simulink model "Multicopter"  (R2018b)
settings: configuration reference "plant_config" (kept outside this file)
values from neighbouring files (symbols this model uses):
  PLANT_EXPORT = Simulink.Parameter(PLANT_EXPORT_VALUE)    [multicopter_model_init.m]    (also in plant_model_init.m)
undefined symbols (not defined in the file or in its folder): acc_x, acc_x_O, acc_y, acc_y_O, acc_z, acc_z_O, alt, alt_ref, day, DiscIntNeverNeededParam, fixType, flags, gSpeed, gyr_x, gyr_y, gyr_z, h_R, hAcc, headAcc, headMot, height, hMSL, hour, iTOW, lat, lat_ref, lon, lon_ref, M_BO, M_OB, mag_x, mag_y, mag_z, month, nano, Newton, numSV, pDOP, phi, PLANT_CONST, plant_model, pressure, prop_vel, psi, quat, Raphson, reserved1, reserved2, rot_x_B, rot_y_B, rot_z_B, sAcc, sec, Sensor_Model, tAcc, temperature, temprature, theta, timestamp, vAcc ... (+10)
libraries: simulink x6, dspsrcs4 x6, AP_Math x3, Rotation x2, Quaternion x2, aerolibatmos2 x1
(part 2 of 2)

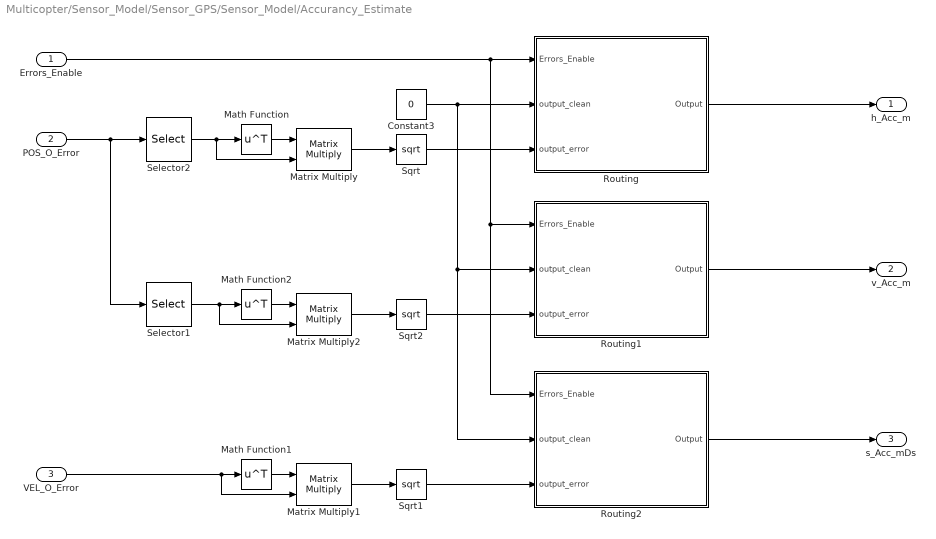
== system Multicopter/Sensor_Model/Sensor_GPS/Sensor_Model/Accurancy_Estimate ==
  Errors_Enable : Inport
  POS_O_Error : Inport  Port=2
  VEL_O_Error : Inport  Port=3
  Constant3 : Constant  Value=0
  Math Function : Math  Operator=transpose  SaturateOnIntegerOverflow=on
  Math Function1 : Math  Operator=transpose  SaturateOnIntegerOverflow=on
  Math Function2 : Math  Operator=transpose  SaturateOnIntegerOverflow=on
  Matrix Multiply : Product  Multiplication=Matrix(*)
  Matrix Multiply1 : Product  Multiplication=Matrix(*)
  Matrix Multiply2 : Product  Multiplication=Matrix(*)
  Routing : Subsystem
  Routing1 : Subsystem
  Routing2 : Subsystem
  Selector1 : Selector  InputPortWidth=3  IndexOptions=Index vector (dialog)  Indices=3  OutputSizes=1
  Selector2 : Selector  InputPortWidth=3  IndexOptions=Index vector (dialog)  Indices=[1 2]  OutputSizes=1
  Sqrt : Sqrt  OutputSignalType=real  SaturateOnIntegerOverflow=on
  Sqrt1 : Sqrt  OutputSignalType=real  SaturateOnIntegerOverflow=on
  Sqrt2 : Sqrt  OutputSignalType=real  SaturateOnIntegerOverflow=on
  h_Acc_m : Outport
  v_Acc_m : Outport  Port=2
  s_Acc_mDs : Outport  Port=3
  wires:
  Sqrt1/1 -> Routing2/3(output_error)
  Routing/1(Output) -> h_Acc_m/1
  Errors_Enable/1 -> Routing2/1(Errors_Enable), Routing1/1(Errors_Enable), Routing/1(Errors_Enable)
  POS_O_Error/1 -> Selector1/1, Selector2/1
  Sqrt/1 -> Routing/3(output_error)
  Constant3/1 -> Routing2/2(output_clean), Routing1/2(output_clean), Routing/2(output_clean)
  Routing1/1(Output) -> v_Acc_m/1
  Selector1/1 -> Math Function2/1, Matrix Multiply2/2
  Routing2/1(Output) -> s_Acc_mDs/1
  Math Function1/1 -> Matrix Multiply1/1
  Math Function2/1 -> Matrix Multiply2/1
  Math Function/1 -> Matrix Multiply/1
  Selector2/1 -> Matrix Multiply/2, Math Function/1
  Matrix Multiply1/1 -> Sqrt1/1
  Sqrt2/1 -> Routing1/3(output_error)
  Matrix Multiply/1 -> Sqrt/1
  Matrix Multiply2/1 -> Sqrt2/1
  VEL_O_Error/1 -> Matrix Multiply1/2, Math Function1/1

== system Multicopter/Sensor_Model/Sensor_GPS/Sensor_Model/GPS_Error ==
  Random Source : dspsrcs4/Random Source  SrcType=Gaussian  NormMethod=Ziggurat  CltLength=12  MinVal=0  MaxVal=1  MeanVal=0  VarVal=[0.02;0.02;0.04].^2  RepMode=Repeatable  rawSeed=1  IsInherit=off  SampMode=Discrete  SampTime=-1  SampFrame=1  DataType=Single  OutComplex=Real  OutputFrames=off
  Random Source1 : dspsrcs4/Random Source  SrcType=Gaussian  NormMethod=Ziggurat  CltLength=12  MinVal=0  MaxVal=1  MeanVal=0  VarVal=[0.01;0.01;0.01].^2  RepMode=Repeatable  rawSeed=1  IsInherit=off  SampMode=Discrete  SampTime=-1  SampFrame=1  DataType=Single  OutComplex=Real  OutputFrames=off
  POS_O_Error : Outport
  VEL_O_Error : Outport  Port=2
  wires:
  Random Source/1 -> POS_O_Error/1
  Random Source1/1 -> VEL_O_Error/1

== system Multicopter/Sensor_Model/Sensor_GPS/Sensor_Model/Routing ==
  Errors_Enable : Inport
  output_clean : Inport  Port=2
  output_error : Inport  Port=3
  Switch : Switch  Criteria=u2 > Threshold
  Output : Outport
  wires:
  output_clean/1 -> Switch/3
  output_error/1 -> Switch/1
  Errors_Enable/1 -> Switch/2
  Switch/1 -> Output/1

== system Multicopter/Sensor_Model/Sensor_GPS/Sensor_Model/Routing1 ==
  Errors_Enable : Inport
  output_clean : Inport  Port=2
  output_error : Inport  Port=3
  Switch : Switch  Criteria=u2 > Threshold
  Output : Outport
  wires:
  Switch/1 -> Output/1
  Errors_Enable/1 -> Switch/2
  output_error/1 -> Switch/1
  output_clean/1 -> Switch/3

== system Multicopter/Sensor_Model/Sensor_GPS/Sensor_Model/WGS84_Linearization ==
  POS_WGS84 : Inport
  POS_O_Error : Inport  Port=2
  Demux2 : Demux  Outputs=3
  Divide2 : Product  Inputs=/*
  Terminator2 : Terminator
  Vector Concatenate2 : Concatenate  NumInputs=3  Mode=Multidimensional array
  WGS84_Linearization : Subsystem  mask{a=6378137, f=1/298.257}
  POS_WGS84_Error : Outport
  wires:
  POS_WGS84/1 -> Demux2/1
  Demux2/1 -> WGS84_Linearization/1(mu_0)
  WGS84_Linearization/2(dy_dlambda) -> Vector Concatenate2/2
  POS_O_Error/1 -> Divide2/2
  Vector Concatenate2/1 -> Divide2/1
  WGS84_Linearization/1(dx_dmu) -> Vector Concatenate2/1
  Demux2/2 -> Terminator2/1
  Demux2/3 -> WGS84_Linearization/2(h_0)
  WGS84_Linearization/3(dz_dh) -> Vector Concatenate2/3
  Divide2/1 -> POS_WGS84_Error/1

== system Multicopter/Sensor_Model/Sensor_GPS/Sensor_Model/pos_filter ==
  POS_WGS84 : Inport
  Discrete FIR Filter : DiscreteFir
  POS_WGS84_meas : Outport
  wires:
  Discrete FIR Filter/1 -> POS_WGS84_meas/1
  POS_WGS84/1 -> Discrete FIR Filter/1

== system Multicopter/Sensor_Model/Sensor_GPS/Sensor_Model/vel_filter ==
  VEL_O : Inport
  Discrete FIR Filter : DiscreteFir
  VEL_O_meas : Outport
  wires:
  Discrete FIR Filter/1 -> VEL_O_meas/1
  VEL_O/1 -> Discrete FIR Filter/1

== system Multicopter/Sensor_Model/Sensor_IMU/Accelerometer/Bus Assignment ==
  Output : Inport
  Bus Creator : BusCreator  Inputs=3
  Demux : Demux  Outputs=3
  Acc_Raw : Outport
  wires:
  Demux/2 -> Bus Creator/2  "Acc_y_mDs2"
  Demux/3 -> Bus Creator/3  "Acc_z_mDs2"
  Demux/1 -> Bus Creator/1  "Acc_x_mDs2"
  Bus Creator/1 -> Acc_Raw/1
  Output/1 -> Demux/1

== system Multicopter/Sensor_Model/Sensor_IMU/Accelerometer/Physical_Model ==
  States : Inport
  Vibration_Enbale : Inport  Port=2
  Routing : Subsystem
  Specific_Force : Subsystem
  Sum1 : Sum  Inputs=|++
  Vibration_Model : Subsystem  TreatAsAtomicUnit=on  mask{Weight=Sensor_Model.Acc.Vibration.Weight, u_max=Sensor_Model.Acc.Vibration.RPM_Max, Gain=Sensor_Model.Acc.Vibration.Gain}
      mask prompts: Weight "input weight"; u_max "max RPM"; Gain "vibration gain"
      mask help: propeller vibration model
      settings: RTWSystemCode=Inline
  prop_vel : Subsystem
  sfor_B_mPs2 : Outport  Unit=m/s^2
  wires:
  States/1 -> prop_vel/1(States), Specific_Force/1(States)
  Routing/1(y) -> sfor_B_mPs2/1
  Sum1/1 -> Routing/3(output_error)
  Vibration_Model/1(vibration) -> Sum1/2
  Vibration_Enbale/1 -> Routing/1(Vibration_Enbale)
  prop_vel/1(omega_radDs) -> Vibration_Model/1(prop_rot_radPs)
  Specific_Force/1(sfor_B_mPs2) -> Routing/2(output_clean), Sum1/1

== system Multicopter/Sensor_Model/Sensor_IMU/Accelerometer/Sensor_Model ==
  Errors_Enables : Inport
  u : Inport  Port=2
  Lowpass_Filter : Subsystem
  Routing : Subsystem
  Saturation : Saturate  UpperLimit=Sensor_Model.Acc.Upper_limit  LowerLimit=Sensor_Model.Acc.Lower_limit
  Sensor_Error : Subsystem
  Sum : Sum  Inputs=|++
  White Noise : Subsystem
  y : Outport
  wires:
  Routing/1(y) -> y/1
  Errors_Enables/1 -> Routing/1(Errors_Enables)
  Sum/1 -> Routing/3(output_error)
  Saturation/1 -> Sum/1
  Lowpass_Filter/1(y) -> Saturation/1
  Sensor_Error/1(y) -> Lowpass_Filter/1(u)
  White Noise/1(noise) -> Sum/2
  u/1 -> Routing/2(output_clean), Sensor_Error/1(u)

== system Multicopter/Sensor_Model/Sensor_IMU/Gyroscope/Bus Assignment ==
  Output : Inport
  Bus Creator : BusCreator  Inputs=3
  Demux : Demux  Outputs=3
  Gyro_Raw : Outport
  wires:
  Demux/1 -> Bus Creator/1  "Gyro_x_radDs"
  Demux/2 -> Bus Creator/2  "Gyro_y_radDs"
  Demux/3 -> Bus Creator/3  "Gyro_z_radDs"
  Bus Creator/1 -> Gyro_Raw/1
  Output/1 -> Demux/1

== system Multicopter/Sensor_Model/Sensor_IMU/Gyroscope/Physical_Model ==
  States : Inport
  Vibration_Enable : Inport  Port=2
  Routing : Subsystem
  Sum : Sum  Inputs=|++
  Vibration_Model : Subsystem  TreatAsAtomicUnit=on  mask{Weight=Sensor_Model.Gyro.Vibration.Weight, u_max=Sensor_Model.Gyro.Vibration.RPM_Max, Gain=Sensor_Model.Gyro.Vibration.Gain}
      mask prompts: Weight "input weight"; u_max "max RPM"; Gain "vibration gain"
      mask help: propeller vibration model
      settings: RTWSystemCode=Inline
  prop_vel : Subsystem
  selection : Subsystem
  gyr_B_radDs : Outport  Unit=rad/s
  wires:
  States/1 -> selection/1(States), prop_vel/1(States)
  selection/1(rot_radPs) -> Sum/1, Routing/2(output_clean)
  Sum/1 -> Routing/3(output_error)
  Vibration_Model/1(vibration) -> Sum/2
  Routing/1(y) -> gyr_B_radDs/1
  Vibration_Enable/1 -> Routing/1(Vibration_Enable)
  prop_vel/1(omega_radPs) -> Vibration_Model/1(prop_rot_radPs)

== system Multicopter/Sensor_Model/Sensor_IMU/Gyroscope/Sensor_Model ==
  Errors_Enable : Inport
  u : Inport  Port=2
  LPF : Subsystem
  Routing : Subsystem
  Saturation : Saturate  UpperLimit=Sensor_Model.Gyro.Range  LowerLimit=-Sensor_Model.Gyro.Range
  Sensor_Error : Subsystem
  Sum : Sum  Inputs=|++
  White Noise : Subsystem
  y : Outport
  wires:
  u/1 -> Routing/2(output_clean), Sensor_Error/1(u)
  Routing/1(y) -> y/1
  Errors_Enable/1 -> Routing/1(Errors_Enable)
  Sum/1 -> Routing/3(output_error)
  Saturation/1 -> Sum/1
  LPF/1(y) -> Saturation/1
  Sensor_Error/1(y) -> LPF/1(u)
  White Noise/1(noise) -> Sum/2

== system Multicopter/Sensor_Model/Sensor_MAG/Sensor_Magnetometer/Bus Assignment ==
  Output : Inport
  Bus Creator : BusCreator  Inputs=3
  Demux : Demux  Outputs=3
  Mag_Raw : Outport
  wires:
  Demux/2 -> Bus Creator/2  "Mag_y_gauss"
  Demux/1 -> Bus Creator/1  "Mag_x_gauss"
  Bus Creator/1 -> Mag_Raw/1
  Demux/3 -> Bus Creator/3  "Mag_z_gauss"
  Output/1 -> Demux/1

== system Multicopter/Sensor_Model/Sensor_MAG/Sensor_Magnetometer/Physical_Model ==
  States : Inport
  Bus Selector : BusSelector  OutputSignals=Plant_States.lat,Plant_States.lon
  Bus Selector1 : BusSelector  OutputSignals=Extended_States.M_BO
  Magnetic_Field : Subsystem
  Product : Product  Multiplication=Matrix(*)  RndMeth=Zero  InputSameDT=on  OutDataTypeStr=Inherit: Same as first input
  wmm_lookup : Subsystem  mask{wmm_magnitude=Sensor_Model.Mag.WMM_Mag, wmm_declination=Sensor_Model.Mag.WMM_Dec, wmm_inclination=Sensor_Model.Mag.WMM_Inc, res=10}
      mask prompts: wmm_magnitude "WMM Magnitude Lookup Table"; wmm_declination "WMM Declination Lookup Table"; wmm_inclination "WMM Inclination Lookup Table"; res "Resolution"
  mag_B_Gauss : Outport  Unit=T  PortDimensions=[3 1]
  wires:
  States/1 -> Bus Selector1/1, Bus Selector/1
  Bus Selector/2 -> wmm_lookup/2(lon_rad)  "<lon>"
  Bus Selector/1 -> wmm_lookup/1(lat_rad)  "<lat>"
  wmm_lookup/1(magnitude_uT) -> Magnetic_Field/1(magnitude_uT)
  wmm_lookup/2(declination_deg) -> Magnetic_Field/2(declination_deg)
  wmm_lookup/3(inclination_deg) -> Magnetic_Field/3(inclination_deg)
  Bus Selector1/1 -> Product/1  "<M_BO>"
  Product/1 -> mag_B_Gauss/1
  Magnetic_Field/1(mag_O_gauss) -> Product/2

== system Multicopter/Sensor_Model/Sensor_MAG/Sensor_Magnetometer/Sensor_Model ==
  Errors_Enable : Inport
  u : Inport  Port=2
  Add : Sum  InputSameDT=on  OutDataTypeStr=Inherit: Same as first input
  Routing : Subsystem
  Saturation : Saturate  UpperLimit=Sensor_Model.Mag.Upper_limit  LowerLimit=Sensor_Model.Mag.Lower_limit
  Sensor_Error : Subsystem
  Signal Conversion1 : SignalConversion  OverrideOpt=on
  White_Noise : Subsystem
  y : Outport
  wires:
  Signal Conversion1/1 -> Routing/2(output_clean)
  Routing/1(y) -> y/1
  Errors_Enable/1 -> Routing/1(Errors_Enable)
  Add/1 -> Routing/3(output_error)
  Saturation/1 -> Add/1
  Sensor_Error/1(y) -> Saturation/1
  u/1 -> Signal Conversion1/1, Sensor_Error/1(u)
  White_Noise/1(noise) -> Add/2

== system Multicopter/Sensor_Model/Sensor_GPS/Sensor_Model/Accurancy_Estimate/Routing ==
  Errors_Enable : Inport
  output_clean : Inport  Port=2
  output_error : Inport  Port=3
  Switch : Switch  Criteria=u2 > Threshold
  Output : Outport
  wires:
  output_clean/1 -> Switch/3
  output_error/1 -> Switch/1
  Errors_Enable/1 -> Switch/2
  Switch/1 -> Output/1

== system Multicopter/Sensor_Model/Sensor_GPS/Sensor_Model/Accurancy_Estimate/Routing1 ==
  Errors_Enable : Inport
  output_clean : Inport  Port=2
  output_error : Inport  Port=3
  Switch : Switch  Criteria=u2 > Threshold
  Output : Outport
  wires:
  Switch/1 -> Output/1
  Errors_Enable/1 -> Switch/2
  output_error/1 -> Switch/1
  output_clean/1 -> Switch/3

== system Multicopter/Sensor_Model/Sensor_GPS/Sensor_Model/Accurancy_Estimate/Routing2 ==
  Errors_Enable : Inport
  output_clean : Inport  Port=2
  output_error : Inport  Port=3
  Switch : Switch  Criteria=u2 > Threshold
  Output : Outport
  wires:
  output_clean/1 -> Switch/3
  output_error/1 -> Switch/1
  Errors_Enable/1 -> Switch/2
  Switch/1 -> Output/1

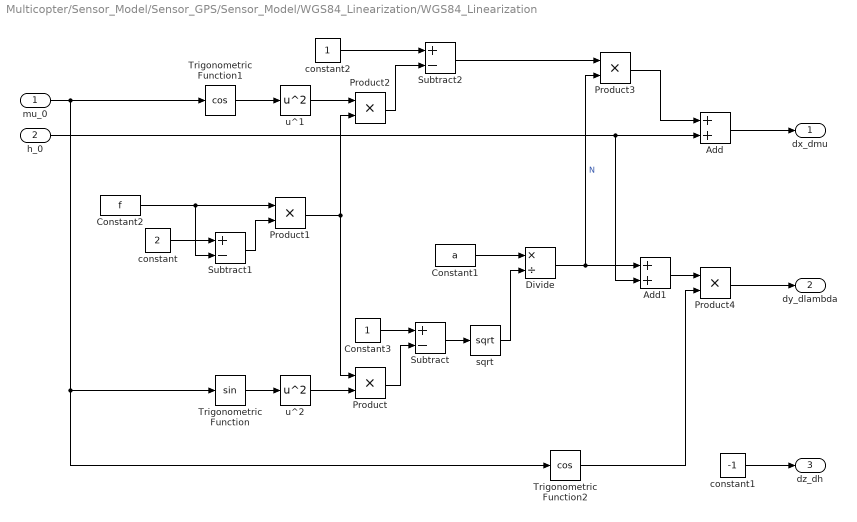
== system Multicopter/Sensor_Model/Sensor_GPS/Sensor_Model/WGS84_Linearization/WGS84_Linearization ==
  mu_0 : Inport
  h_0 : Inport  Port=2
  Add : Sum
  Add1 : Sum
  Constant1 : Constant  Value=a
  Constant2 : Constant  Value=f
  Constant3 : Constant
  Divide : Product  Inputs=*/
  Product{,1..4} (5 alike) : Product  RndMeth=Zero
  Subtract : Sum  Inputs=+-
  Subtract1 : Sum  Inputs=+-
  Subtract2 : Sum  Inputs=+-
  Trigonometric Function : Trigonometry
  Trigonometric Function1 : Trigonometry  Operator=cos
  Trigonometric Function2 : Trigonometry  Operator=cos
  constant : Constant  Value=2
  constant1 : Constant  Value=-1
  constant2 : Constant
  sqrt : Sqrt  AlgorithmType=Newton-Raphson  SaturateOnIntegerOverflow=on
  u^1 : Math  Operator=square  SaturateOnIntegerOverflow=on
  u^2 : Math  Operator=square  SaturateOnIntegerOverflow=on
  dx_dmu : Outport
  dy_dlambda : Outport  Port=2
  dz_dh : Outport  Port=3
  wires:
  Product4/1 -> dy_dlambda/1
  Add1/1 -> Product4/1
  Trigonometric Function2/1 -> Product4/2
  Product3/1 -> Add/1
  Subtract2/1 -> Product3/1
  Product2/1 -> Subtract2/2
  u^1/1 -> Product2/1
  Trigonometric Function1/1 -> u^1/1
  constant2/1 -> Subtract2/1
  h_0/1 -> Add1/2, Add/2
  Add/1 -> dx_dmu/1
  constant1/1 -> dz_dh/1
  Divide/1 -> Add1/1, Product3/2  "N"
  sqrt/1 -> Divide/2
  Product1/1 -> Product2/2, Product/1
  Subtract1/1 -> Product1/2
  constant/1 -> Subtract1/1
  Constant2/1 -> Subtract1/2, Product1/1
  Product/1 -> Subtract/2
  Subtract/1 -> sqrt/1
  Constant3/1 -> Subtract/1
  u^2/1 -> Product/2
  Trigonometric Function/1 -> u^2/1
  mu_0/1 -> Trigonometric Function2/1, Trigonometric Function/1, Trigonometric Function1/1
  Constant1/1 -> Divide/1

== system Multicopter/Sensor_Model/Sensor_IMU/Accelerometer/Physical_Model/Routing ==
  Vibration_Enbale : Inport
  output_clean : Inport  Port=2
  output_error : Inport  Port=3
  Switch : Switch  Criteria=u2 > Threshold  OutDataTypeStr=single
  y : Outport
  wires:
  Vibration_Enbale/1 -> Switch/2
  output_clean/1 -> Switch/3
  output_error/1 -> Switch/1
  Switch/1 -> y/1

== system Multicopter/Sensor_Model/Sensor_IMU/Accelerometer/Physical_Model/Specific_Force ==
  States : Inport
  Bus Selector : BusSelector  OutputSignals=Plant_States.acc_x_O,Plant_States.acc_y_O,Plant_States.acc_z_O
  Bus Selector1 : BusSelector  OutputSignals=Extended_States.M_BO
  Gravity : Constant  Value=[0;0;Sensor_Model.g]  OutDataTypeStr=single
  Product1 : Product  Multiplication=Matrix(*)  RndMeth=Zero  InputSameDT=on  OutDataTypeStr=Inherit: Same as first input
  Sum : Sum  Inputs=|+-  InputSameDT=on  OutDataTypeStr=Inherit: Same as first input
  Vector Concatenate1 : Concatenate  NumInputs=3  Mode=Multidimensional array
  sfor_B_mPs2 : Outport  Unit=m/s^2
  wires:
  States/1 -> Bus Selector1/1, Bus Selector/1
  Bus Selector/1 -> Vector Concatenate1/1  "<acc_x_O>"
  Bus Selector/2 -> Vector Concatenate1/2  "<acc_y_O>"
  Bus Selector/3 -> Vector Concatenate1/3  "<acc_z_O>"
  Product1/1 -> sfor_B_mPs2/1
  Bus Selector1/1 -> Product1/1  "<M_BO>"
  Vector Concatenate1/1 -> Sum/1
  Sum/1 -> Product1/2
  Gravity/1 -> Sum/2

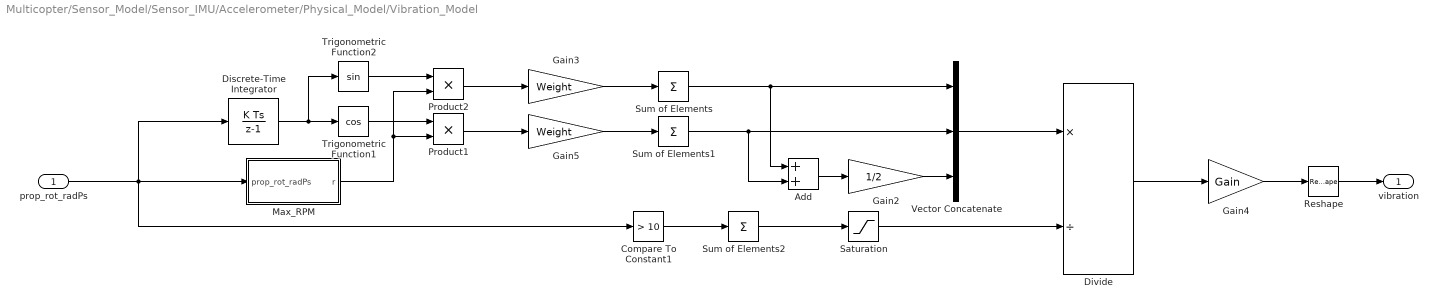
== system Multicopter/Sensor_Model/Sensor_IMU/Accelerometer/Physical_Model/Vibration_Model ==
  prop_rot_radPs : Inport  PortDimensions=[4,1]
  Add : Sum
  Compare To Constant1 : simulink/Logic and Bit Operations/Compare To Constant  relop=>  const=10  OutDataTypeStr=boolean
  Discrete-Time Integrator : DiscreteIntegrator  InitialCondition=zeros(4,1)  SampleTime=-1  ICPrevOutput=DiscIntNeverNeededParam  ICPrevScaledInput=DiscIntNeverNeededParam
  Divide : Product  Inputs=*/
  Gain2 : Gain  Gain=1/2
  Gain3 : Gain  Gain=Weight
  Gain4 : Gain  Gain=Gain
  Gain5 : Gain  Gain=Weight
  Max_RPM : Subsystem
  Product1 : Product  RndMeth=Zero
  Product2 : Product  RndMeth=Zero
  Reshape : Reshape  OutputDimensionality=Column vector (2-D)
  Saturation : Saturate  UpperLimit=8  LowerLimit=4
  Sum of Elements : Sum  Inputs=+
  Sum of Elements1 : Sum  Inputs=+
  Sum of Elements2 : Sum  Inputs=+  CollapseMode=Specified dimension
  Trigonometric Function1 : Trigonometry  Operator=cos
  Trigonometric Function2 : Trigonometry
  Vector Concatenate : Concatenate  NumInputs=3  Mode=Multidimensional array
  vibration : Outport
  wires:
  prop_rot_radPs/1 -> Discrete-Time Integrator/1, Compare To Constant1/1, Max_RPM/1(prop_rot_radPs)
  Sum of Elements2/1 -> Saturation/1
  Saturation/1 -> Divide/2
  Divide/1 -> Gain4/1
  Compare To Constant1/1 -> Sum of Elements2/1
  Vector Concatenate/1 -> Divide/1
  Product1/1 -> Gain5/1
  Trigonometric Function1/1 -> Product1/1
  Product2/1 -> Gain3/1
  Trigonometric Function2/1 -> Product2/1
  Gain2/1 -> Vector Concatenate/3
  Add/1 -> Gain2/1
  Sum of Elements1/1 -> Add/2, Vector Concatenate/2
  Discrete-Time Integrator/1 -> Trigonometric Function2/1, Trigonometric Function1/1
  Sum of Elements/1 -> Add/1, Vector Concatenate/1
  Reshape/1 -> vibration/1
  Gain3/1 -> Sum of Elements/1
  Gain5/1 -> Sum of Elements1/1
  Gain4/1 -> Reshape/1
  Max_RPM/1(r) -> Product1/2, Product2/2

== system Multicopter/Sensor_Model/Sensor_IMU/Accelerometer/Physical_Model/prop_vel ==
  States : Inport
  Bus Selector2 : BusSelector  OutputSignals=Extended_States.prop_vel
  Selector : Selector  InputPortWidth=8  IndexOptions=Index vector (dialog)  Indices=[1:4]  OutputSizes=1
  omega_radDs : Outport
  wires:
  States/1 -> Bus Selector2/1
  Bus Selector2/1 -> Selector/1  "<prop_vel>"
  Selector/1 -> omega_radDs/1

== system Multicopter/Sensor_Model/Sensor_IMU/Accelerometer/Sensor_Model/Lowpass_Filter ==
  u : Inport
  Constant : Constant  Value=2*pi*Sensor_Model.Acc.Cutoff_frequency_Hz  VectorParams1D=off  OutDataTypeStr=single
  Product : Product  RndMeth=Zero  InputSameDT=on  OutDataTypeStr=Inherit: Same as first input
  Product1 : Product  RndMeth=Zero  InputSameDT=on  OutDataTypeStr=Inherit: Same as first input
  Sum : Sum  Inputs=|+-  InputSameDT=on  OutDataTypeStr=Inherit: Same as first input
  Sum1 : Sum  Inputs=|+-  InputSameDT=on  OutDataTypeStr=Inherit: Same as first input
  integrate : DiscreteIntegrator  SampleTime=-1  ICPrevOutput=DiscIntNeverNeededParam  ICPrevScaledInput=DiscIntNeverNeededParam
  integrate1 : DiscreteIntegrator  SampleTime=-1  ICPrevOutput=DiscIntNeverNeededParam  ICPrevScaledInput=DiscIntNeverNeededParam
  y : Outport
  wires:
  integrate1/1 -> Sum1/2, y/1
  Product1/1 -> integrate1/1
  Sum1/1 -> Product1/2
  integrate/1 -> Sum/2, Sum1/1
  Product/1 -> integrate/1
  Constant/1 -> Product1/1, Product/1
  Sum/1 -> Product/2
  u/1 -> Sum/1

== system Multicopter/Sensor_Model/Sensor_IMU/Accelerometer/Sensor_Model/Routing ==
  Errors_Enables : Inport
  output_clean : Inport  Port=2
  output_error : Inport  Port=3
  Switch : Switch  Criteria=u2 > Threshold
  y : Outport
  wires:
  Switch/1 -> y/1
  output_error/1 -> Switch/1
  output_clean/1 -> Switch/3
  Errors_Enables/1 -> Switch/2

== system Multicopter/Sensor_Model/Sensor_IMU/Accelerometer/Sensor_Model/Sensor_Error ==
  u : Inport
  Add : Sum  InputSameDT=on  OutDataTypeStr=Inherit: Same as first input
  Constant : Constant  Value=eye(3)  OutDataTypeStr=single
  Constant1 : Constant  Value=Sensor_Model.Acc.Scalefactor_Error  VectorParams1D=off  OutDataTypeStr=single
  Constant3 : Constant  Value=Sensor_Model.Acc.Bias  VectorParams1D=off  OutDataTypeStr=single
  Product : Product  Multiplication=Matrix(*)  RndMeth=Zero  InputSameDT=on  OutDataTypeStr=Inherit: Same as first input
  Sum : Sum  Inputs=|++  InputSameDT=on  OutDataTypeStr=Inherit: Same as first input
  y : Outport
  wires:
  Sum/1 -> y/1
  Add/1 -> Product/1
  u/1 -> Product/2
  Constant1/1 -> Add/2
  Constant/1 -> Add/1
  Product/1 -> Sum/1
  Constant3/1 -> Sum/2

== system Multicopter/Sensor_Model/Sensor_IMU/Accelerometer/Sensor_Model/White Noise ==
  Random Source : dspsrcs4/Random Source  SrcType=Gaussian  NormMethod=Ziggurat  CltLength=12  MinVal=0  MaxVal=1  MeanVal=0  VarVal=Sensor_Model.Acc.Variance  RepMode=Repeatable  rawSeed=1  IsInherit=off  SampMode=Discrete  SampTime=-1  SampFrame=1  DataType=Single  OutComplex=Real  OutputFrames=off
  noise : Outport
  wires:
  Random Source/1 -> noise/1

== system Multicopter/Sensor_Model/Sensor_IMU/Gyroscope/Physical_Model/Routing ==
  Vibration_Enable : Inport
  output_clean : Inport  Port=2
  output_error : Inport  Port=3
  Switch : Switch  Criteria=u2 > Threshold
  y : Outport
  wires:
  Vibration_Enable/1 -> Switch/2
  output_clean/1 -> Switch/3
  output_error/1 -> Switch/1
  Switch/1 -> y/1

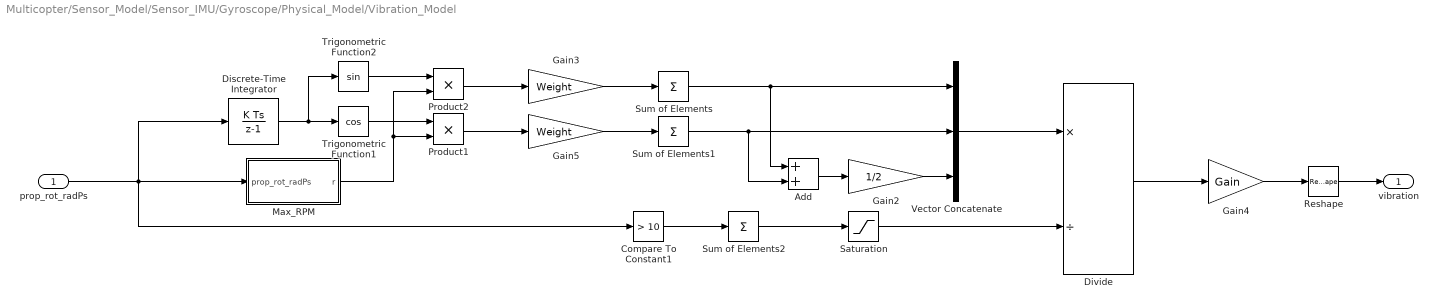
== system Multicopter/Sensor_Model/Sensor_IMU/Gyroscope/Physical_Model/Vibration_Model ==
  prop_rot_radPs : Inport  PortDimensions=[4,1]
  Add : Sum
  Compare To Constant1 : simulink/Logic and Bit Operations/Compare To Constant  relop=>  const=10  OutDataTypeStr=boolean
  Discrete-Time Integrator : DiscreteIntegrator  InitialCondition=zeros(4,1)  SampleTime=-1  ICPrevOutput=DiscIntNeverNeededParam  ICPrevScaledInput=DiscIntNeverNeededParam
  Divide : Product  Inputs=*/
  Gain2 : Gain  Gain=1/2
  Gain3 : Gain  Gain=Weight
  Gain4 : Gain  Gain=Gain
  Gain5 : Gain  Gain=Weight
  Max_RPM : Subsystem
  Product1 : Product  RndMeth=Zero
  Product2 : Product  RndMeth=Zero
  Reshape : Reshape  OutputDimensionality=Column vector (2-D)
  Saturation : Saturate  UpperLimit=8  LowerLimit=4
  Sum of Elements : Sum  Inputs=+
  Sum of Elements1 : Sum  Inputs=+
  Sum of Elements2 : Sum  Inputs=+  CollapseMode=Specified dimension
  Trigonometric Function1 : Trigonometry  Operator=cos
  Trigonometric Function2 : Trigonometry
  Vector Concatenate : Concatenate  NumInputs=3  Mode=Multidimensional array
  vibration : Outport
  wires:
  prop_rot_radPs/1 -> Discrete-Time Integrator/1, Compare To Constant1/1, Max_RPM/1(prop_rot_radPs)
  Sum of Elements2/1 -> Saturation/1
  Saturation/1 -> Divide/2
  Divide/1 -> Gain4/1
  Compare To Constant1/1 -> Sum of Elements2/1
  Vector Concatenate/1 -> Divide/1
  Product1/1 -> Gain5/1
  Trigonometric Function1/1 -> Product1/1
  Product2/1 -> Gain3/1
  Trigonometric Function2/1 -> Product2/1
  Gain2/1 -> Vector Concatenate/3
  Add/1 -> Gain2/1
  Sum of Elements1/1 -> Add/2, Vector Concatenate/2
  Discrete-Time Integrator/1 -> Trigonometric Function2/1, Trigonometric Function1/1
  Sum of Elements/1 -> Add/1, Vector Concatenate/1
  Reshape/1 -> vibration/1
  Gain3/1 -> Sum of Elements/1
  Gain5/1 -> Sum of Elements1/1
  Gain4/1 -> Reshape/1
  Max_RPM/1(r) -> Product1/2, Product2/2

== system Multicopter/Sensor_Model/Sensor_IMU/Gyroscope/Physical_Model/prop_vel ==
  States : Inport
  Bus Selector2 : BusSelector  OutputSignals=Extended_States.prop_vel
  Selector : Selector  InputPortWidth=8  IndexOptions=Index vector (dialog)  Indices=[1:4]  OutputSizes=1
  omega_radPs : Outport
  wires:
  Selector/1 -> omega_radPs/1
  States/1 -> Bus Selector2/1
  Bus Selector2/1 -> Selector/1  "<prop_vel>"

== system Multicopter/Sensor_Model/Sensor_IMU/Gyroscope/Physical_Model/selection ==
  States : Inport
  Bus Selector2 : BusSelector  OutputSignals=Plant_States.rot_x_B,Plant_States.rot_y_B,Plant_States.rot_z_B
  Vector Concatenate : Concatenate  NumInputs=3  Mode=Multidimensional array
  rot_radPs : Outport
  wires:
  Vector Concatenate/1 -> rot_radPs/1
  Bus Selector2/3 -> Vector Concatenate/3  "<rot_z_B>"
  Bus Selector2/1 -> Vector Concatenate/1  "<rot_x_B>"
  Bus Selector2/2 -> Vector Concatenate/2  "<rot_y_B>"
  States/1 -> Bus Selector2/1

== system Multicopter/Sensor_Model/Sensor_IMU/Gyroscope/Sensor_Model/LPF ==
  u : Inport
  Constant : Constant  Value=2*pi*Sensor_Model.Gyro.Cutoff_frequency_Hz  VectorParams1D=off  OutDataTypeStr=single
  Product : Product  RndMeth=Zero  InputSameDT=on  OutDataTypeStr=Inherit: Same as first input
  Product1 : Product  RndMeth=Zero  InputSameDT=on  OutDataTypeStr=Inherit: Same as first input
  Sum : Sum  Inputs=|+-  InputSameDT=on  OutDataTypeStr=Inherit: Same as first input
  Sum1 : Sum  Inputs=|+-  InputSameDT=on  OutDataTypeStr=Inherit: Same as first input
  integrate : DiscreteIntegrator  SampleTime=-1  ICPrevOutput=DiscIntNeverNeededParam  ICPrevScaledInput=DiscIntNeverNeededParam
  integrate1 : DiscreteIntegrator  SampleTime=-1  ICPrevOutput=DiscIntNeverNeededParam  ICPrevScaledInput=DiscIntNeverNeededParam
  y : Outport
  wires:
  integrate1/1 -> Sum1/2, y/1
  Product1/1 -> integrate1/1
  Sum1/1 -> Product1/2
  integrate/1 -> Sum/2, Sum1/1
  Product/1 -> integrate/1
  Constant/1 -> Product1/1, Product/1
  Sum/1 -> Product/2
  u/1 -> Sum/1

== system Multicopter/Sensor_Model/Sensor_IMU/Gyroscope/Sensor_Model/Routing ==
  Errors_Enable : Inport
  output_clean : Inport  Port=2
  output_error : Inport  Port=3
  Switch : Switch  Criteria=u2 > Threshold
  y : Outport
  wires:
  Switch/1 -> y/1
  output_error/1 -> Switch/1
  output_clean/1 -> Switch/3
  Errors_Enable/1 -> Switch/2

== system Multicopter/Sensor_Model/Sensor_IMU/Gyroscope/Sensor_Model/Sensor_Error ==
  u : Inport
  Add : Sum  InputSameDT=on  OutDataTypeStr=Inherit: Same as first input
  Constant1 : Constant  Value=Sensor_Model.Gyro.Scalefactor_Error  VectorParams1D=off  OutDataTypeStr=single
  Constant2 : Constant  Value=eye(3)  OutDataTypeStr=single
  Constant3 : Constant  Value=Sensor_Model.Gyro.Bias  VectorParams1D=off  OutDataTypeStr=single
  Product : Product  Multiplication=Matrix(*)  RndMeth=Zero  InputSameDT=on  OutDataTypeStr=Inherit: Same as first input
  Sum : Sum  Inputs=|++  InputSameDT=on  OutDataTypeStr=Inherit: Same as first input
  y : Outport
  wires:
  Sum/1 -> y/1
  Product/1 -> Sum/1
  u/1 -> Product/2
  Add/1 -> Product/1
  Constant1/1 -> Add/2
  Constant2/1 -> Add/1
  Constant3/1 -> Sum/2

== system Multicopter/Sensor_Model/Sensor_IMU/Gyroscope/Sensor_Model/White Noise ==
  Random Source : dspsrcs4/Random Source  SrcType=Gaussian  NormMethod=Ziggurat  CltLength=12  MinVal=0  MaxVal=1  MeanVal=0  VarVal=Sensor_Model.Gyro.Variance  RepMode=Repeatable  rawSeed=1  IsInherit=off  SampMode=Discrete  SampTime=-1  SampFrame=1  DataType=Single  OutComplex=Real  OutputFrames=off
  noise : Outport
  wires:
  Random Source/1 -> noise/1

== system Multicopter/Sensor_Model/Sensor_MAG/Sensor_Magnetometer/Physical_Model/Magnetic_Field ==
  magnitude_uT : Inport
  declination_deg : Inport  Port=2
  inclination_deg : Inport  Port=3
  Constant : Constant  Value=[1;0;0]  OutDataTypeStr=single
  Gain : Gain  Gain=-pi/180
  Gain1 : Gain  Gain=pi/180
  Gain2 : Gain  Gain=0.01
  Multiply : Product
  Multiply1 : Product  Multiplication=Matrix(*)
  Multiply2 : Product  Multiplication=Matrix(*)
  Rot_y to M : Subsystem
  Rot_z to M : Subsystem
  mag_O_gauss : Outport
  wires:
  Constant/1 -> Multiply/2
  Multiply/1 -> Multiply1/2  "mag_field"
  Rot_y to M/1(My) -> Multiply1/1
  inclination_deg/1 -> Gain/1
  Gain/1 -> Rot_y to M/1(alpha)
  declination_deg/1 -> Gain1/1
  Gain1/1 -> Rot_z to M/1(alpha)
  Rot_z to M/1(Mz) -> Multiply2/1
  magnitude_uT/1 -> Gain2/1
  Gain2/1 -> Multiply/1  "magnitude_gauss"
  Multiply1/1 -> Multiply2/2
  Multiply2/1 -> mag_O_gauss/1

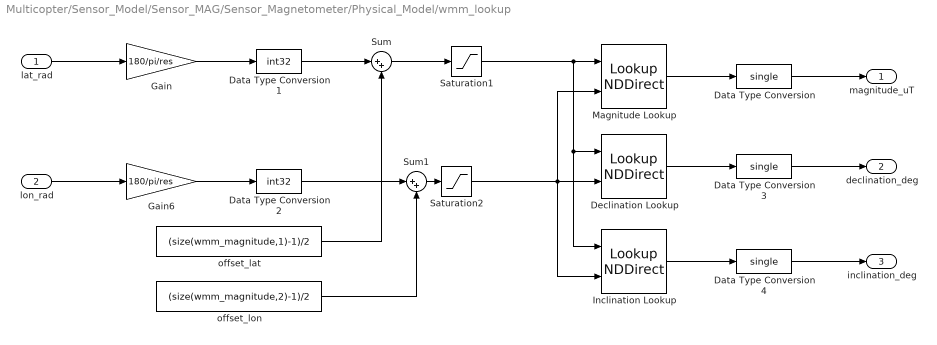
== system Multicopter/Sensor_Model/Sensor_MAG/Sensor_Magnetometer/Physical_Model/wmm_lookup ==
  lat_rad : Inport
  lon_rad : Inport  Port=2
  Data Type Conversion : DataTypeConversion  OutDataTypeStr=single
  Data Type Conversion1 : DataTypeConversion  OutDataTypeStr=int32  RndMeth=Simplest
  Data Type Conversion2 : DataTypeConversion  OutDataTypeStr=int32  RndMeth=Simplest
  Data Type Conversion3 : DataTypeConversion  OutDataTypeStr=single
  Data Type Conversion4 : DataTypeConversion  OutDataTypeStr=single
  Declination Lookup : LookupNDDirect  Table=wmm_declination  TableDataTypeStr=int16
  Gain : Gain  Gain=180/pi/res
  Gain6 : Gain  Gain=180/pi/res
  Inclination Lookup : LookupNDDirect  Table=wmm_inclination  TableDataTypeStr=int8
  Magnitude Lookup : LookupNDDirect  Table=wmm_magnitude  TableDataTypeStr=uint8
  Saturation1 : Saturate  UpperLimit=size(wmm_magnitude,1)-1  LowerLimit=0
  Saturation2 : Saturate  UpperLimit=size(wmm_magnitude,2)-1  LowerLimit=0
  Sum : Sum  Inputs=|++
  Sum1 : Sum  Inputs=|++
  offset_lat : Constant  Value=(size(wmm_magnitude,1)-1)/2  OutDataTypeStr=int32
  offset_lon : Constant  Value=(size(wmm_magnitude,2)-1)/2  OutDataTypeStr=int32
  magnitude_uT : Outport
  declination_deg : Outport  Port=2
  inclination_deg : Outport  Port=3
  wires:
  Data Type Conversion4/1 -> inclination_deg/1
  Inclination Lookup/1 -> Data Type Conversion4/1
  Data Type Conversion3/1 -> declination_deg/1
  Data Type Conversion/1 -> magnitude_uT/1
  offset_lon/1 -> Sum1/2
  offset_lat/1 -> Sum/2
  Sum1/1 -> Saturation2/1
  Gain6/1 -> Data Type Conversion2/1
  Sum/1 -> Saturation1/1
  Gain/1 -> Data Type Conversion1/1
  Saturation2/1 -> Magnitude Lookup/2, Declination Lookup/2, Inclination Lookup/2
  Saturation1/1 -> Magnitude Lookup/1, Declination Lookup/1, Inclination Lookup/1
  Magnitude Lookup/1 -> Data Type Conversion/1
  Declination Lookup/1 -> Data Type Conversion3/1
  lat_rad/1 -> Gain/1
  lon_rad/1 -> Gain6/1
  Data Type Conversion1/1 -> Sum/1
  Data Type Conversion2/1 -> Sum1/1

== system Multicopter/Sensor_Model/Sensor_MAG/Sensor_Magnetometer/Sensor_Model/Routing ==
  Errors_Enable : Inport
  output_clean : Inport  Port=2
  output_error : Inport  Port=3
  Switch : Switch  Criteria=u2 > Threshold
  y : Outport
  wires:
  Switch/1 -> y/1
  output_error/1 -> Switch/1
  output_clean/1 -> Switch/3
  Errors_Enable/1 -> Switch/2

== system Multicopter/Sensor_Model/Sensor_MAG/Sensor_Magnetometer/Sensor_Model/Sensor_Error ==
  u : Inport
  Add : Sum  InputSameDT=on  OutDataTypeStr=Inherit: Same as first input
  Constant : Constant  Value=eye(3)  OutDataTypeStr=single
  Constant1 : Constant  Value=Sensor_Model.Mag.Scalefactor_Error  VectorParams1D=off  OutDataTypeStr=single
  Constant3 : Constant  Value=Sensor_Model.Mag.Bias  VectorParams1D=off  OutDataTypeStr=single
  Product : Product  Multiplication=Matrix(*)  RndMeth=Zero  InputSameDT=on  OutDataTypeStr=Inherit: Same as first input
  Sum : Sum  Inputs=|++  InputSameDT=on  OutDataTypeStr=Inherit: Same as first input
  y : Outport
  wires:
  Sum/1 -> y/1
  Constant/1 -> Add/1
  Product/1 -> Sum/1
  u/1 -> Product/2
  Constant1/1 -> Add/2
  Add/1 -> Product/1
  Constant3/1 -> Sum/2

== system Multicopter/Sensor_Model/Sensor_MAG/Sensor_Magnetometer/Sensor_Model/White_Noise ==
  Random Source : dspsrcs4/Random Source  SrcType=Gaussian  NormMethod=Ziggurat  CltLength=12  MinVal=0  MaxVal=1  MeanVal=0  VarVal=Sensor_Model.Mag.Variance  RepMode=Repeatable  rawSeed=1  IsInherit=off  SampMode=Discrete  SampTime=-1  SampFrame=1  DataType=Single  OutComplex=Real  OutputFrames=off
  noise : Outport
  wires:
  Random Source/1 -> noise/1

== system Multicopter/Sensor_Model/Sensor_IMU/Accelerometer/Physical_Model/Vibration_Model/Max_RPM ==
  prop_rot_radPs : Inport
  Constant : Constant  Value=u_max  VectorParams1D=off
  Constant1 : Constant  Value=30  VectorParams1D=off
  Divide1 : Product  Inputs=*/
  Divide2 : Product  Inputs=*/
  Gain6 : Gain  Gain=pi
  u^2 : Math  Operator=square  SaturateOnIntegerOverflow=on
  r : Outport
  wires:
  Divide2/1 -> u^2/1
  prop_rot_radPs/1 -> Divide2/1
  Constant/1 -> Gain6/1
  Divide1/1 -> Divide2/2
  Gain6/1 -> Divide1/1
  u^2/1 -> r/1
  Constant1/1 -> Divide1/2

== system Multicopter/Sensor_Model/Sensor_IMU/Gyroscope/Physical_Model/Vibration_Model/Max_RPM ==
  prop_rot_radPs : Inport
  Constant : Constant  Value=u_max  VectorParams1D=off
  Constant1 : Constant  Value=30  VectorParams1D=off
  Divide1 : Product  Inputs=*/
  Divide2 : Product  Inputs=*/
  Gain6 : Gain  Gain=pi
  u^2 : Math  Operator=square  SaturateOnIntegerOverflow=on
  r : Outport
  wires:
  Divide2/1 -> u^2/1
  prop_rot_radPs/1 -> Divide2/1
  Constant/1 -> Gain6/1
  Divide1/1 -> Divide2/2
  Gain6/1 -> Divide1/1
  u^2/1 -> r/1
  Constant1/1 -> Divide1/2

== system Multicopter/Sensor_Model/Sensor_MAG/Sensor_Magnetometer/Physical_Model/Magnetic_Field/Rot_y to M ==
  alpha : Inport
  Constant{,2..4} (4 alike) : Constant  Value=0  OutDataTypeStr=Inherit: Inherit via back propagation
  Constant1 : Constant  OutDataTypeStr=Inherit: Inherit via back propagation
  Gain1 : Gain  Gain=-1
  Trigonometric Function : Trigonometry
  Trigonometric Function1 : Trigonometry  Operator=cos
  Trigonometric Function2 : Trigonometry
  Trigonometric Function3 : Trigonometry  Operator=cos
  Vector Concatenate : Concatenate  NumInputs=3  Mode=Multidimensional array  ConcatenateDimension=2
  Vector Concatenate1 : Concatenate  NumInputs=3  Mode=Multidimensional array
  Vector Concatenate2 : Concatenate  NumInputs=3  Mode=Multidimensional array
  Vector Concatenate3 : Concatenate  NumInputs=3  Mode=Multidimensional array
  My : Outport
  wires:
  alpha/1 -> Trigonometric Function3/1, Trigonometric Function2/1, Trigonometric Function/1, Trigonometric Function1/1
  Constant4/1 -> Vector Concatenate2/2
  Trigonometric Function3/1 -> Vector Concatenate2/3
  Trigonometric Function2/1 -> Vector Concatenate2/1
  Trigonometric Function/1 -> Gain1/1
  Trigonometric Function1/1 -> Vector Concatenate1/1
  Constant/1 -> Vector Concatenate3/3
  Constant1/1 -> Vector Concatenate3/2
  Constant2/1 -> Vector Concatenate3/1
  Vector Concatenate3/1 -> Vector Concatenate/2
  Vector Concatenate2/1 -> Vector Concatenate/3
  Vector Concatenate1/1 -> Vector Concatenate/1
  Vector Concatenate/1 -> My/1
  Constant3/1 -> Vector Concatenate1/2
  Gain1/1 -> Vector Concatenate1/3

== system Multicopter/Sensor_Model/Sensor_MAG/Sensor_Magnetometer/Physical_Model/Magnetic_Field/Rot_z to M ==
  alpha : Inport
  Constant : Constant  OutDataTypeStr=Inherit: Inherit via back propagation
  Constant{1..4} (4 alike) : Constant  Value=0  OutDataTypeStr=Inherit: Inherit via back propagation
  Gain : Gain  Gain=-1
  Trigonometric Function : Trigonometry
  Trigonometric Function1 : Trigonometry  Operator=cos
  Trigonometric Function2 : Trigonometry
  Trigonometric Function3 : Trigonometry  Operator=cos
  Vector Concatenate : Concatenate  NumInputs=3  Mode=Multidimensional array  ConcatenateDimension=2
  Vector Concatenate1 : Concatenate  NumInputs=3  Mode=Multidimensional array
  Vector Concatenate2 : Concatenate  NumInputs=3  Mode=Multidimensional array
  Vector Concatenate3 : Concatenate  NumInputs=3  Mode=Multidimensional array
  Mz : Outport
  wires:
  alpha/1 -> Trigonometric Function3/1, Trigonometric Function2/1, Trigonometric Function/1, Trigonometric Function1/1
  Constant4/1 -> Vector Concatenate2/3
  Trigonometric Function3/1 -> Vector Concatenate2/2
  Gain/1 -> Vector Concatenate2/1
  Trigonometric Function2/1 -> Gain/1
  Constant3/1 -> Vector Concatenate1/3
  Trigonometric Function/1 -> Vector Concatenate1/2
  Trigonometric Function1/1 -> Vector Concatenate1/1
  Constant/1 -> Vector Concatenate3/3
  Constant1/1 -> Vector Concatenate3/2
  Constant2/1 -> Vector Concatenate3/1
  Vector Concatenate3/1 -> Vector Concatenate/3
  Vector Concatenate2/1 -> Vector Concatenate/2
  Vector Concatenate1/1 -> Vector Concatenate/1
  Vector Concatenate/1 -> Mz/1
